simulink model "sampleModel2044"  (R2023a)
settings: Solver=VariableStepAuto  StartTime=0.0  StopTime=10.0  RelTol=1e-3
libraries: hdlsllib x5
settings Model: Creator=user1  LastModifiedBy=user1

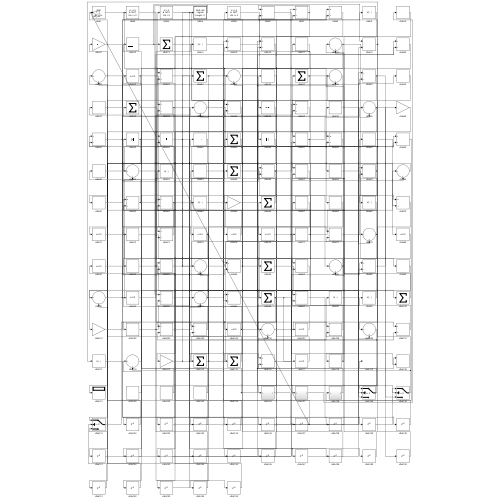
[thumbnail: Simulink's stored preview of the top-level diagram]
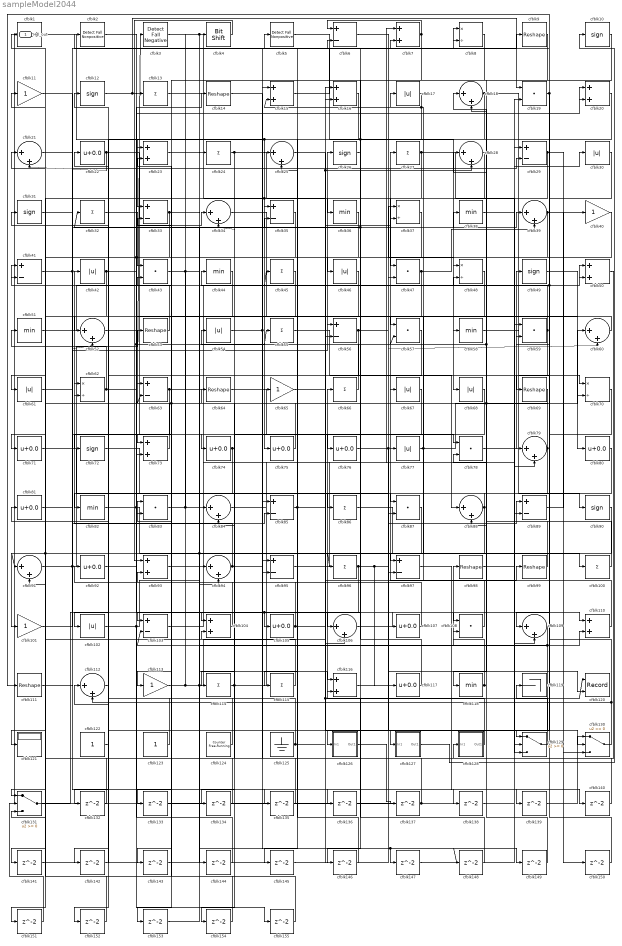
== system sampleModel2044 ==
  cfblk1 : ArithShift  BitShiftNumber=8
  cfblk{10,12,26,31,49,72,90} (7 alike) : Signum
  cfblk{13,24,27,32,45,55,66,86,96,100,114..115} (12 alike) : Sum  Inputs=+  OutDataTypeStr=uint8
  cfblk{11,40,65,101,113} (5 alike) : Gain  OutDataTypeStr=uint8
  cfblk{17,30,42,46,54,61,67..68,77,102} (10 alike) : Abs  OutDataTypeStr=uint8  SaturateOnIntegerOverflow=off
  cfblk{6,29,33,35,41,56,63,85,89,95,97,103} (12 alike) : Sum  Inputs=+-  OutDataTypeStr=uint8
  cfblk{7,15..16,20,23,50,73,93,104,110,116} (11 alike) : Sum  OutDataTypeStr=uint8
  cfblk{22,71,74..76,80..81,92,105,107,117} (11 alike) : Bias  Bias=0.0  SaturateOnIntegerOverflow=off
  cfblk{18,21,25,28,34,39,52,60,79,84,88,91,94,106,109,112} (16 alike) : Sum  Inputs=|++  OutDataTypeStr=uint8
  cfblk{19,43,47,57,59,78,83,87,108} (9 alike) : DotProduct  OutDataTypeStr=uint8
  cfblk{9,14,53,64,69,98..99,111} (8 alike) : Reshape
  cfblk{36,38,44,51,58,82,118} (7 alike) : MinMax  OutDataTypeStr=uint8
  cfblk119 : Terminator
  cfblk120 : Record  FileSettingsInternal="{\"entries\":[{\"content\":{\"excelSettings\":{\"content\":{},\"type\":\"Streamout.ExcelSettings\"}},\"type\":\"Streamout.FileSettingStorage\",\"uuid\":\"\"}],\"packageUris\":[\"http:\\/\\/schema.mathworks.com\\/mf0\\/streamout_blocks\\/R2020a\"],\"version\":\"1.0\"}"  Layout=[1 1]  SignalsInternal="{\"entries\":[{\"content\":{\"signals\":[{\"content\":{\"blockPath\":[],\"dimensions\":[1],\"domain\":\"\",\"lineColor\":\"#a2142f\",\"plots\":[1],\"port\":1,\"signalID\":59982,\"signalName\":\"cfblk125\"},\"type\":\"RecordBlkView.Signal\",\"uuid\":\"\"},{\"content\":{\"blockPath\":[],\"dimensions\":[1],\"domain\":\"\",\"lineColor\":\"#139fff\",\"plots\":[1],\"port\":2,\"signalID\":59985,\"signalName\":\"cfblk96\"},\"type\":\"RecordBlkView.Signal\",\"uuid\":\"\"}]},\"type\":\"RecordBlkView.InputSignals\",\"uuid\":\"\"}],\"packageUris\":[\"http:\\/\\/schema.mathworks.com\\/mf0\\/streamout_blocks\\/R2020a\"],\"version\":\"1.0\"}"  VisualizationBindings="{\"xyplotplugin\":{\"info\":[{\"series\":[{\"bindingParametersList\":[{\"parameter\":\"X-Axis\",\"signalID\":59982,\"signalName\":\"cfblk125\"},{\"parameter\":\"Y-Axis\",\"signalID\":59985,\"signalName\":\"cfblk96\"}],\"seriesID\":18060}],\"subplotID\":1}]}}"  CompatibilityTag=XY  st=-1
  cfblk121 : Display
  cfblk122 : Constant  OutDataTypeStr=uint8  SampleTime=-1
  cfblk123 : Constant  OutDataTypeStr=uint8  SampleTime=-1
  cfblk124 : hdlsllib/Sources/Counter Free-Running  NumBits=16  tsamp=-1
  cfblk125 : Ground
  cfblk126 : Subsystem
      settings: LibrarySourceBlock=|
      | hdlsllib/Ports &
      | Subsystems/Subsystem
  cfblk127 : Subsystem
      settings: LibrarySourceBlock=|
      | hdlsllib/Ports &
      | Subsystems/Subsystem
  cfblk128 : Subsystem
      settings: LibrarySourceBlock=|
      | hdlsllib/Ports &
      | Subsystems/Subsystem
  cfblk129 : Switch  OutDataTypeStr=uint8  SaturateOnIntegerOverflow=off  InputSameDT=off
  cfblk130 : Switch  OutDataTypeStr=uint8  SaturateOnIntegerOverflow=off  InputSameDT=off
  cfblk131 : Switch  OutDataTypeStr=uint8  SaturateOnIntegerOverflow=off  InputSameDT=off
  cfblk{132..155} (24 alike) : Delay  SampleTime=1
  cfblk2 : hdlsllib/Logic and Bit Operations/Detect Fall Nonpositive  vinit=0  OutDataTypeStr=uint8
  cfblk3 : hdlsllib/Logic and Bit Operations/Detect Fall Negative  vinit=0  OutDataTypeStr=uint8
  cfblk{8,37,48,62,70} (5 alike) : Product  Inputs=*/  OutDataTypeStr=uint8  RndMeth=Zero  SaturateOnIntegerOverflow=on
  cfblk4 : hdlsllib/Logic and Bit Operations/Bit Shift  mode=Shift Left Logical  N=0
  cfblk5 : hdlsllib/Logic and Bit Operations/Detect Fall Nonpositive  vinit=0  OutDataTypeStr=uint8
  Hdl_out : Outport  OutDataTypeStr=uint8
  wires:
  cfblk75/1 -> cfblk3/1, cfblk23/2
  cfblk66/1 -> cfblk26/1
  cfblk96/1 -> cfblk105/1, cfblk143/1, cfblk117/1, cfblk120/2
  cfblk4/1 -> cfblk93/1
  cfblk109/1 -> cfblk103/2, cfblk142/1
  cfblk89/1 -> cfblk40/1
  cfblk108/1 -> cfblk27/1
  cfblk114/1 -> cfblk7/1, cfblk64/1
  cfblk95/1 -> cfblk77/1
  cfblk60/1 -> cfblk57/1
  cfblk110/1 -> cfblk67/1
  cfblk128/1(Out1) -> cfblk66/1
  cfblk103/1 -> cfblk50/1
  cfblk40/1 -> cfblk68/1
  cfblk50/1 -> cfblk128/1(In1)
  cfblk105/1 -> cfblk93/2, cfblk20/1
  cfblk94/1 -> cfblk42/1, cfblk8/2
  cfblk12/1 -> cfblk19/1, cfblk87/2
  cfblk29/1 -> cfblk75/1, cfblk71/1, cfblk150/1
  cfblk73/1 -> cfblk22/1
  cfblk62/1 -> cfblk51/1, cfblk35/2
  cfblk15/1 -> cfblk7/2
  cfblk19/1 -> cfblk111/1, cfblk69/1
  cfblk74/1 -> cfblk153/1, cfblk154/1
  cfblk26/1 -> cfblk126/1(In1)
  cfblk92/1 -> cfblk55/1, cfblk14/1
  cfblk22/1 -> cfblk76/1, cfblk21/2
  cfblk131/1 -> cfblk104/1
  cfblk118/1 -> cfblk98/1, cfblk78/2
  cfblk32/1 -> cfblk43/1
  cfblk106/1 -> cfblk108/1
  cfblk124/1 -> cfblk31/1
  cfblk104/1 -> cfblk83/1
  cfblk129/1 -> cfblk119/1
  cfblk47/1 -> cfblk131/1, cfblk39/2
  cfblk91/1 -> cfblk53/1, cfblk56/1
  cfblk58/1 -> cfblk70/1
  cfblk34/1 -> cfblk80/1
  cfblk18/1 -> cfblk90/1, cfblk65/1
  cfblk2/1 -> cfblk13/1
  cfblk122/1 -> cfblk62/1
  cfblk39/1 -> cfblk82/1, cfblk73/2, cfblk130/3
  cfblk36/1 -> cfblk73/1
  cfblk42/1 -> cfblk56/2, cfblk151/1
  cfblk123/1 -> cfblk81/1
  cfblk49/1 -> cfblk70/2
  cfblk28/1 -> cfblk47/1
  cfblk99/1 -> cfblk54/1, cfblk63/2
  cfblk88/1 -> cfblk86/1, cfblk132/1
  cfblk77/1 -> cfblk60/1, cfblk17/1
  cfblk48/1 -> cfblk97/1
  cfblk25/1 -> cfblk127/1(In1), cfblk28/2
  cfblk63/1 -> cfblk15/1, cfblk72/1
  cfblk115/1 -> cfblk11/1
  cfblk17/1 -> cfblk35/1, cfblk52/1, cfblk15/2
  cfblk72/1 -> cfblk107/1
  cfblk80/1 -> cfblk102/1
  cfblk78/1 -> cfblk49/1
  cfblk5/1 -> cfblk58/1
  cfblk57/1 -> cfblk115/1
  cfblk100/1 -> cfblk44/1, cfblk57/2
  cfblk79/1 -> cfblk118/1, cfblk21/1
  cfblk61/1 -> cfblk8/1
  cfblk35/1 -> cfblk113/1
  cfblk68/1 -> cfblk106/1
  cfblk14/1 -> cfblk147/1, cfblk148/1
  cfblk21/1 -> cfblk74/1
  cfblk54/1 -> cfblk50/2, cfblk138/1
  cfblk90/1 -> cfblk101/1
  cfblk41/1 -> cfblk39/1, cfblk52/2
  cfblk43/1 -> cfblk100/1, cfblk84/1
  cfblk51/1 -> cfblk29/1
  cfblk102/1 -> cfblk38/1, cfblk20/2, cfblk155/1
  cfblk16/1 -> cfblk33/1
  cfblk69/1 -> cfblk62/2
  cfblk53/1 -> cfblk41/1
  cfblk27/1 -> cfblk79/2, cfblk84/2
  cfblk59/1 -> cfblk18/1, cfblk87/1
  cfblk8/1 -> cfblk36/1
  cfblk82/1 -> cfblk34/1, cfblk109/2
  cfblk23/1 -> cfblk96/1, cfblk140/1
  cfblk113/1 -> cfblk99/1, cfblk110/2, cfblk4/1
  cfblk83/1 -> cfblk16/1, cfblk24/1
  cfblk70/1 -> cfblk129/1
  cfblk30/1 -> cfblk109/1
  cfblk117/1 -> cfblk32/1, cfblk6/2
  cfblk84/1 -> cfblk30/1
  cfblk65/1 -> cfblk37/2
  cfblk85/1 -> cfblk5/1, cfblk97/2
  cfblk13/1 -> cfblk85/1
  cfblk76/1 -> cfblk129/2, cfblk60/2
  cfblk101/1 -> cfblk9/1
  cfblk6/1 -> cfblk48/1
  cfblk81/1 -> cfblk85/2
  cfblk127/1(Out1) -> cfblk10/1
  cfblk67/1 -> cfblk114/1
  cfblk24/1 -> cfblk106/2, cfblk34/2
  cfblk20/1 -> cfblk145/1, cfblk146/1
  cfblk116/1 -> cfblk89/1
  cfblk125/1 -> cfblk120/1, cfblk108/2, cfblk43/2
  cfblk33/1 -> cfblk116/1, cfblk61/1
  cfblk7/1 -> cfblk6/1, cfblk23/1
  cfblk130/1 -> cfblk45/1, cfblk2/1, cfblk112/2
  cfblk86/1 -> cfblk129/3
  cfblk31/1 -> cfblk29/2
  cfblk38/1 -> cfblk130/2
  cfblk55/1 -> cfblk88/1
  cfblk56/1 -> cfblk48/2, cfblk152/1
  cfblk107/1 -> cfblk92/1
  cfblk3/1 -> cfblk95/2, cfblk149/1
  cfblk64/1 -> cfblk78/1
  cfblk46/1 -> cfblk91/1, cfblk121/1
  cfblk37/1 -> cfblk46/1
  cfblk71/1 -> cfblk94/2
  cfblk10/1 -> cfblk88/2
  cfblk98/1 -> cfblk59/1
  cfblk1/1 -> cfblk25/1
  cfblk112/1 -> cfblk12/1
  cfblk87/1 -> cfblk103/1
  cfblk52/1 -> cfblk110/1
  cfblk132/1 -> cfblk1/1
  cfblk9/1 -> cfblk133/1
  cfblk133/1 -> cfblk89/2
  cfblk45/1 -> cfblk134/1
  cfblk134/1 -> cfblk33/2
  cfblk111/1 -> cfblk135/1
  cfblk135/1 -> cfblk104/2
  cfblk11/1 -> cfblk136/1
  cfblk136/1 -> cfblk79/1
  cfblk126/1(Out1) -> cfblk137/1
  cfblk137/1 -> cfblk41/2, Hdl_out/1
  cfblk138/1 -> cfblk18/2
  cfblk97/1 -> cfblk139/1
  cfblk139/1 -> cfblk130/1
  cfblk140/1 -> cfblk95/1
  cfblk44/1 -> cfblk141/1
  cfblk141/1 -> cfblk37/1
  cfblk142/1 -> cfblk112/1
  cfblk143/1 -> cfblk16/2
  cfblk93/1 -> cfblk144/1
  cfblk144/1 -> cfblk63/1
  cfblk145/1 -> cfblk47/2
  cfblk146/1 -> cfblk25/2
  cfblk147/1 -> cfblk19/2
  cfblk148/1 -> cfblk116/2
  cfblk149/1 -> cfblk28/1
  cfblk150/1 -> cfblk59/2
  cfblk151/1 -> cfblk131/2
  cfblk152/1 -> cfblk131/3
  cfblk153/1 -> cfblk94/1
  cfblk154/1 -> cfblk83/2
  cfblk155/1 -> cfblk91/2

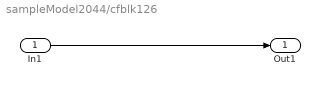
== system sampleModel2044/cfblk126 ==
  In1 : Inport
  Out1 : Outport
  wires:
  In1/1 -> Out1/1

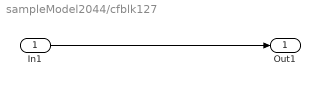
== system sampleModel2044/cfblk127 ==
  In1 : Inport
  Out1 : Outport
  wires:
  In1/1 -> Out1/1

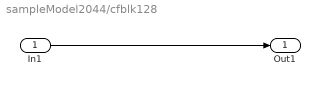
== system sampleModel2044/cfblk128 ==
  In1 : Inport
  Out1 : Outport
  wires:
  In1/1 -> Out1/1
